simulink model "model"  (R2015b)
settings: Solver=VariableStepAuto  StartTime=0.0  StopTime=20  MaxStep=0.01  RelTol=1e-8
settings Model: Creator=Pracownik  LastModifiedBy=DarekP

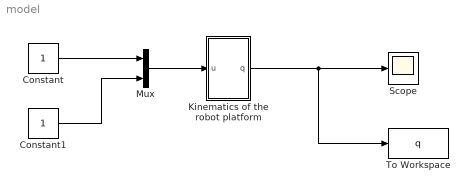
== system model ==
  Constant : Constant
  Constant1 : Constant
  Kinematics of the robot platform : Subsystem
  Mux : Mux  Inputs=2
  Scope : Scope
  To Workspace : ToWorkspace  VariableName=q  SampleTime=-1
  wires:
  Kinematics of the robot platform/1(q) -> To Workspace/1, Scope/1
  Mux/1 -> Kinematics of the robot platform/1(u)
  Constant/1 -> Mux/1
  Constant1/1 -> Mux/2

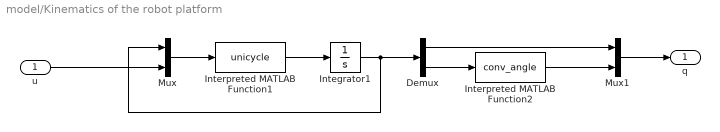
== system model/Kinematics of the robot platform ==
  u : Inport
  Demux : Demux  Outputs=[2 1]
  Integrator1 : Integrator  InitialCondition=[0; 0; 0]
  Interpreted MATLAB Function1 : MATLABFcn  MATLABFcn=unicycle
  Interpreted MATLAB Function2 : MATLABFcn  MATLABFcn=conv_angle
  Mux : Mux  Inputs=[3 2]
  Mux1 : Mux  Inputs=[2 1]
  q : Outport
  wires:
  Mux/1 -> Interpreted MATLAB Function1/1
  Interpreted MATLAB Function1/1 -> Integrator1/1
  Integrator1/1 -> Demux/1, Mux/1
  u/1 -> Mux/2
  Demux/2 -> Interpreted MATLAB Function2/1
  Interpreted MATLAB Function2/1 -> Mux1/2
  Demux/1 -> Mux1/1
  Mux1/1 -> q/1
